simulink model "RFSwPFC"  (R2024a)
settings: Solver=VariableStepAuto  StartTime=0.0  StopTime=0.1  RelTol=1e-3
undefined symbols (not defined in the file or in its folder): bE, c, vr, wg
libraries: cstblocks x3
settings Model: Creator=FactCore  LastModifiedBy=FactCore

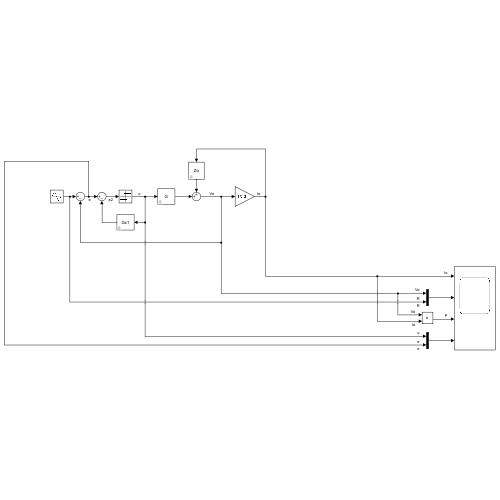
[thumbnail: Simulink's stored preview of the top-level diagram]
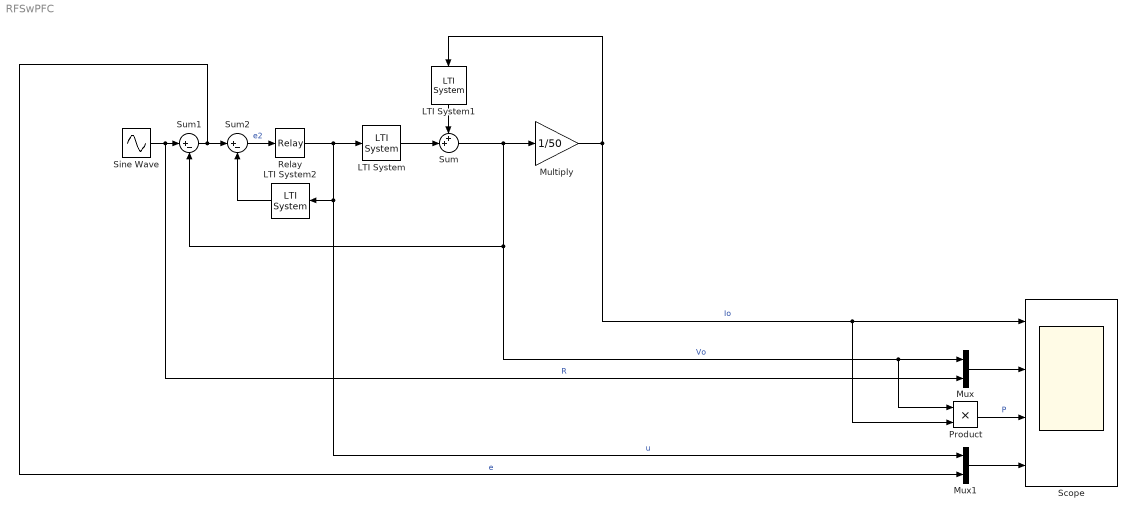
== system RFSwPFC ==
  LTI System : cstblocks/LTI System  sys=G  IC=[]  PadeOrder=0
  LTI System1 : cstblocks/LTI System  sys=Zo  IC=[]  PadeOrder=0
  LTI System2 : cstblocks/LTI System  sys=Gc1  IC=[]  PadeOrder=0
  Multiply : Gain  Gain=1/50
  Mux : Mux  Inputs=2
  Mux1 : Mux  Inputs=2
  Product : Product
  Relay : Relay  OnSwitchValue=bE  OffSwitchValue=-bE  OnOutputValue=c  OffOutputValue=-c
  Scope : Scope  NumInputPorts=4
  Sine Wave : Sin  Amplitude=vr*sqrt(2)  Frequency=wg  SampleTime=0
  Sum : Sum  Inputs=++|
  Sum1 : Sum  Inputs=|+-
  Sum2 : Sum  Inputs=|+-
  wires:
  Multiply/1 -> Product/2, Scope/1, LTI System1/1  "Io"
  Mux/1 -> Scope/2
  Mux1/1 -> Scope/4
  LTI System1/1 -> Sum/1
  Sum1/1 -> Sum2/1, Mux1/2  "e"
  Sine Wave/1 -> Mux/2, Sum1/1  "R"
  Relay/1 -> LTI System2/1, Mux1/1, LTI System/1  "u"
  Product/1 -> Scope/3  "P"
  LTI System/1 -> Sum/2
  Sum/1 -> Multiply/1, Product/1, Mux/1, Sum1/2  "Vo"
  Sum2/1 -> Relay/1  "e2"
  LTI System2/1 -> Sum2/2
